simulink model "c2dModel"  (R2017a)
settings: Solver=VariableStepAuto  StartTime=0.0  StopTime=10.0  RelTol=1e-3
values from neighbouring files (symbols this model uses):
  dden = cell2mat(dsys.Denominator)    [exmM_IM.m]    (also in tmp3.m)
  den = [1 3 10]    [exmM_IM.m]    (also in tmp3.m)
  dnum = cell2mat(dsys.Numerator)    [exmM_IM.m]    (also in tmp3.m)
  num = 10    [exmM_IM.m]    (also in tmp3.m)
  Ts = 0.1    [exmM_IM.m]    (also in tmp3.m)
settings Model: Creator=lzr96  LastModifiedBy=lzr96

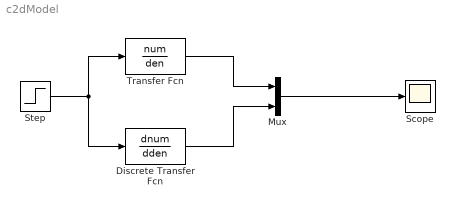
== system c2dModel ==
  Discrete Transfer Fcn : DiscreteTransferFcn  Numerator=dnum  Denominator=dden  SampleTime=Ts
  Mux : Mux  Inputs=3
  Scope : Scope
  Step : Step  SampleTime=0
  Transfer Fcn : TransferFcn  Numerator=num  Denominator=den
  wires:
  Step/1 -> Discrete Transfer Fcn/1, Transfer Fcn/1
  Transfer Fcn/1 -> Mux/1
  Discrete Transfer Fcn/1 -> Mux/3
  Mux/1 -> Scope/1
